simulink model "Problem_2"  (R2020a)
settings: Solver=VariableStepAuto  StartTime=0.0  StopTime=100  RelTol=1e-3
undefined symbols (not defined in the file): b, k1, m1
settings Model: Creator=Ganesh  LastModifiedBy=Avengers
settings DataIOCC: ExternalInput=[t, stin]  LoadExternalInput=on  SaveFormat=Structure

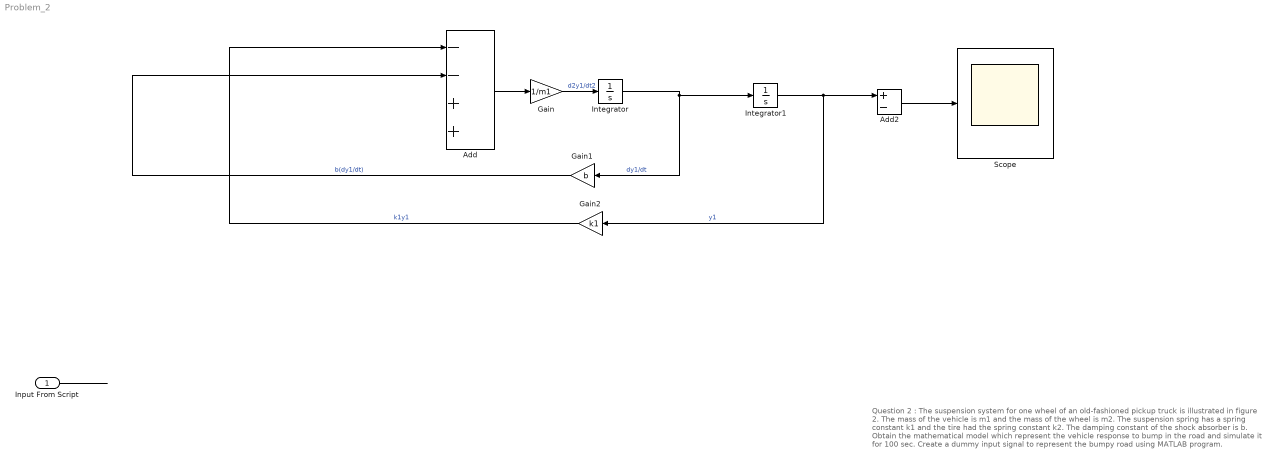
== system Problem_2 ==
  note: Question 2 : The suspension system for one wheel of an old-fashioned pickup truck is illustrated in figure 2. The mass of the vehicle is m1 and the mass of the wheel is m2. The suspension spring has a spring constant k1 and the tire had the spring constant k2. The damping constant of the shock absorber is b. Obtain the mathematical model which represent the vehicle response to bump in the road and simulate it for 100 sec. Create a dummy input signal to represent the bumpy road using MATLAB program.
  Input From Script : Inport
  Add : Sum  Inputs=--++
  Add2 : Sum  Inputs=+-
  Gain : Gain  Gain=1/m1
  Gain1 : Gain  Gain=b
  Gain2 : Gain  Gain=k1
  Integrator : Integrator
  Integrator1 : Integrator
  Scope : Scope
  wires:
  Add/1 -> Gain/1
  Gain/1 -> Integrator/1  "d2y1/dt2"
  Integrator/1 -> Integrator1/1, Gain1/1  "dy1/dt"
  Integrator1/1 -> Add2/1, Gain2/1  "y1"
  Gain1/1 -> Add/2  "b(dy1/dt)"
  Input From Script/1 -> ?
  Gain2/1 -> Add/1  "k1y1"
  Add2/1 -> Scope/1
